simulink model "SignalProcessing"  (R2024a)
settings: Solver=VariableStepAuto  StartTime=0.0  StopTime=1  RelTol=1e-3
undefined symbols (not defined in the file): Fs
libraries: dspfdesign x1
settings Model: Creator=prat  LastModifiedBy=prat
settings DataIOCC: ExternalInput=[t, power]  LoadExternalInput=on

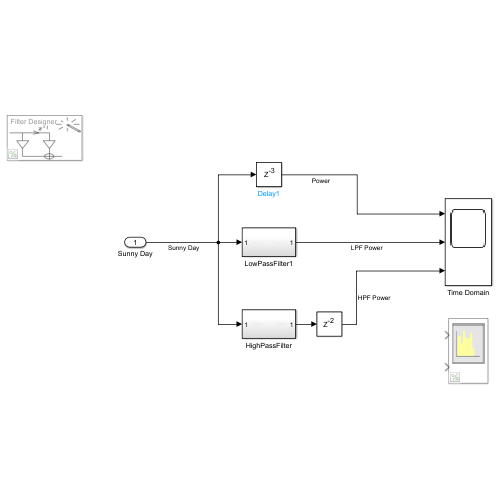
[thumbnail: Simulink's stored preview of the top-level diagram]
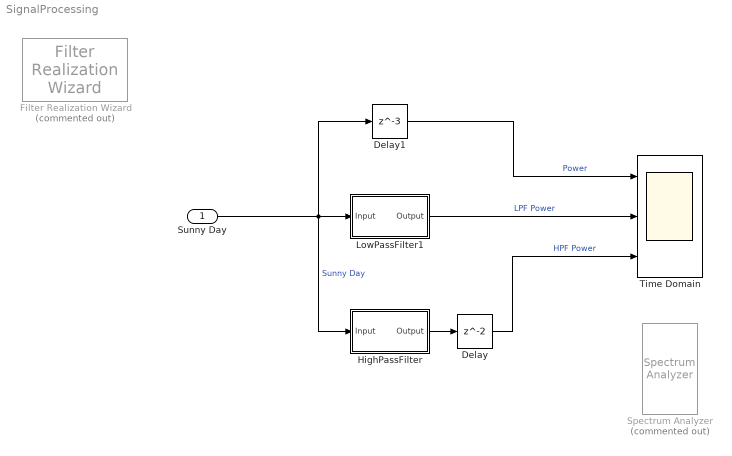
== system SignalProcessing ==
  Sunny Day : Inport  SampleTime=1/Fs
  Delay : Delay
  Delay1 : Delay  DelayLength=3
  Filter Realization Wizard : dspfdesign/Filter Realization Wizard  Commented=on
  HighPassFilter : Subsystem  Tag=FilterWizardSubSystem
      settings: ErrorFcn=dspFilterRealizedInBasicElemsAlgLoopErrFcnCallback
  LowPassFilter1 : Subsystem  Tag=FilterWizardSubSystem
      settings: ErrorFcn=dspFilterRealizedInBasicElemsAlgLoopErrFcnCallback
  Spectrum Analyzer : SpectrumAnalyzer  Commented=on  NumInputPorts=2  WindowPosition=[473.000000,64.000000,800.000000,500.000000,]  ScopeFrameLocation=window  SampleRateSource=Property  SampleRate=44.1e3  PlotAsTwoSidedSpectrum=off  FrequencyScale=Log  FrequencySpan=Start and stop frequencies  StartFrequency=20  StopFrequency=20e3
  Time Domain : Scope  NumInputPorts=3
  wires:
  Sunny Day/1 -> Delay1/1, HighPassFilter/1(Input), LowPassFilter1/1(Input)  "Sunny Day"
  LowPassFilter1/1(Output) -> Time Domain/2  "LPF Power"
  HighPassFilter/1(Output) -> Delay/1
  Delay/1 -> Time Domain/3  "HPF Power"
  Delay1/1 -> Time Domain/1  "Power"

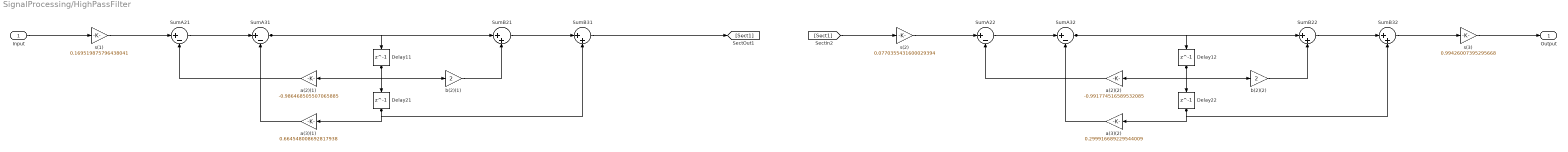
== system SignalProcessing/HighPassFilter ==
  Input : Inport
  Delay{11..12,21..22} (4 alike) : Delay  DelayLength=1  InitialCondition=0
  SumA{21..22,31..32} (4 alike) : Sum  Inputs=|+-  RndMeth=Nearest  SaturateOnIntegerOverflow=on  OutDataTypeStr=Inherit: Same as first input
  SumB{21..22,31..32} (4 alike) : Sum  Inputs=|++  RndMeth=Nearest  SaturateOnIntegerOverflow=on  OutDataTypeStr=Inherit: Same as first input
  a(2)(1) : Gain  Gain=-0.986468505507065885  ParamDataTypeStr=double  RndMeth=Nearest  SaturateOnIntegerOverflow=on  OutDataTypeStr=Inherit: Same as input
  a(2)(2) : Gain  Gain=-0.991774516589532085  ParamDataTypeStr=double  RndMeth=Nearest  SaturateOnIntegerOverflow=on  OutDataTypeStr=Inherit: Same as input
  a(3)(1) : Gain  Gain=0.664548008692817938  ParamDataTypeStr=double  RndMeth=Nearest  SaturateOnIntegerOverflow=on  OutDataTypeStr=Inherit: Same as input
  a(3)(2) : Gain  Gain=0.299916689229544009  ParamDataTypeStr=double  RndMeth=Nearest  SaturateOnIntegerOverflow=on  OutDataTypeStr=Inherit: Same as input
  b(2)(1) : Gain  Gain=2  ParamDataTypeStr=double  RndMeth=Nearest  SaturateOnIntegerOverflow=on  OutDataTypeStr=Inherit: Same as input
  b(2)(2) : Gain  Gain=2  ParamDataTypeStr=double  RndMeth=Nearest  SaturateOnIntegerOverflow=on  OutDataTypeStr=Inherit: Same as input
  s(1) : Gain  Gain=0.169519875796438041  ParamDataTypeStr=double  RndMeth=Nearest  SaturateOnIntegerOverflow=on  OutDataTypeStr=Inherit: Same as input
  s(2) : Gain  Gain=0.0770355431600029394  ParamDataTypeStr=double  RndMeth=Nearest  SaturateOnIntegerOverflow=on  OutDataTypeStr=Inherit: Same as input
  s(3) : Gain  Gain=0.99426007395295668  ParamDataTypeStr=double  RndMeth=Nearest  SaturateOnIntegerOverflow=on  OutDataTypeStr=Inherit: Same as input
  Output : Outport
  wires:
  Input/1 -> s(1)/1
  s(1)/1 -> SumA21/1
  SumA21/1 -> SumA31/1
  SumA31/1 -> SumB21/1, Delay11/1
  SumB21/1 -> SumB31/1
  SumB31/1 -> [Sect1]
  a(2)(1)/1 -> SumA21/2
  Delay11/1 -> a(2)(1)/1, b(2)(1)/1, Delay21/1
  b(2)(1)/1 -> SumB21/2
  a(3)(1)/1 -> SumA31/2
  Delay21/1 -> a(3)(1)/1, SumB31/2
  [Sect1] -> s(2)/1
  s(2)/1 -> SumA22/1
  SumA22/1 -> SumA32/1
  SumA32/1 -> SumB22/1, Delay12/1
  SumB22/1 -> SumB32/1
  SumB32/1 -> s(3)/1
  a(2)(2)/1 -> SumA22/2
  Delay12/1 -> a(2)(2)/1, b(2)(2)/1, Delay22/1
  b(2)(2)/1 -> SumB22/2
  a(3)(2)/1 -> SumA32/2
  Delay22/1 -> a(3)(2)/1, SumB32/2
  s(3)/1 -> Output/1

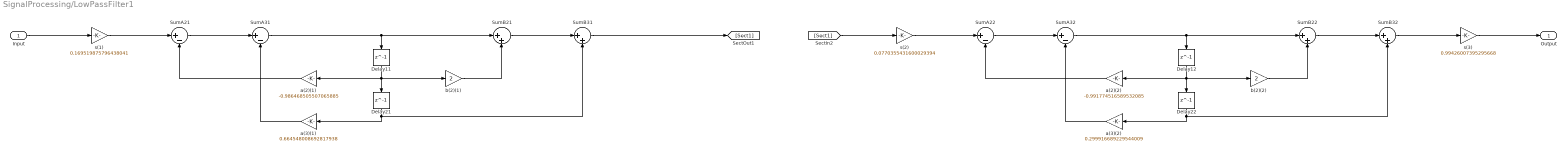
== system SignalProcessing/LowPassFilter1 ==
  Input : Inport
  Delay{11..12,21..22} (4 alike) : Delay  DelayLength=1  InitialCondition=0
  SumA{21..22,31..32} (4 alike) : Sum  Inputs=|+-  RndMeth=Nearest  SaturateOnIntegerOverflow=on  OutDataTypeStr=Inherit: Same as first input
  SumB{21..22,31..32} (4 alike) : Sum  Inputs=|++  RndMeth=Nearest  SaturateOnIntegerOverflow=on  OutDataTypeStr=Inherit: Same as first input
  a(2)(1) : Gain  Gain=-0.986468505507065885  ParamDataTypeStr=double  RndMeth=Nearest  SaturateOnIntegerOverflow=on  OutDataTypeStr=Inherit: Same as input
  a(2)(2) : Gain  Gain=-0.991774516589532085  ParamDataTypeStr=double  RndMeth=Nearest  SaturateOnIntegerOverflow=on  OutDataTypeStr=Inherit: Same as input
  a(3)(1) : Gain  Gain=0.664548008692817938  ParamDataTypeStr=double  RndMeth=Nearest  SaturateOnIntegerOverflow=on  OutDataTypeStr=Inherit: Same as input
  a(3)(2) : Gain  Gain=0.299916689229544009  ParamDataTypeStr=double  RndMeth=Nearest  SaturateOnIntegerOverflow=on  OutDataTypeStr=Inherit: Same as input
  b(2)(1) : Gain  Gain=2  ParamDataTypeStr=double  RndMeth=Nearest  SaturateOnIntegerOverflow=on  OutDataTypeStr=Inherit: Same as input
  b(2)(2) : Gain  Gain=2  ParamDataTypeStr=double  RndMeth=Nearest  SaturateOnIntegerOverflow=on  OutDataTypeStr=Inherit: Same as input
  s(1) : Gain  Gain=0.169519875796438041  ParamDataTypeStr=double  RndMeth=Nearest  SaturateOnIntegerOverflow=on  OutDataTypeStr=Inherit: Same as input
  s(2) : Gain  Gain=0.0770355431600029394  ParamDataTypeStr=double  RndMeth=Nearest  SaturateOnIntegerOverflow=on  OutDataTypeStr=Inherit: Same as input
  s(3) : Gain  Gain=0.99426007395295668  ParamDataTypeStr=double  RndMeth=Nearest  SaturateOnIntegerOverflow=on  OutDataTypeStr=Inherit: Same as input
  Output : Outport
  wires:
  s(3)/1 -> Output/1
  Delay22/1 -> SumB32/2, a(3)(2)/1
  a(3)(2)/1 -> SumA32/2
  b(2)(2)/1 -> SumB22/2
  Delay12/1 -> Delay22/1, b(2)(2)/1, a(2)(2)/1
  a(2)(2)/1 -> SumA22/2
  SumB32/1 -> s(3)/1
  SumB22/1 -> SumB32/1
  SumA32/1 -> Delay12/1, SumB22/1
  SumA22/1 -> SumA32/1
  s(2)/1 -> SumA22/1
  [Sect1] -> s(2)/1
  Delay21/1 -> SumB31/2, a(3)(1)/1
  a(3)(1)/1 -> SumA31/2
  b(2)(1)/1 -> SumB21/2
  Delay11/1 -> Delay21/1, b(2)(1)/1, a(2)(1)/1
  a(2)(1)/1 -> SumA21/2
  SumB31/1 -> [Sect1]
  SumB21/1 -> SumB31/1
  SumA31/1 -> Delay11/1, SumB21/1
  SumA21/1 -> SumA31/1
  s(1)/1 -> SumA21/1
  Input/1 -> s(1)/1
